simulink model "Q53"  (R2023a)
settings: Solver=VariableStepAuto  StartTime=0.0  StopTime=10.0  MaxStep=0.001  RelTol=1e-3
settings Model: Creator=Physics Library  LastModifiedBy=Physics Library

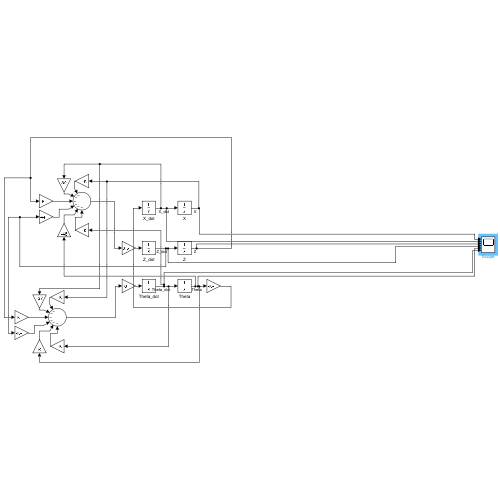
[thumbnail: Simulink's stored preview of the top-level diagram]
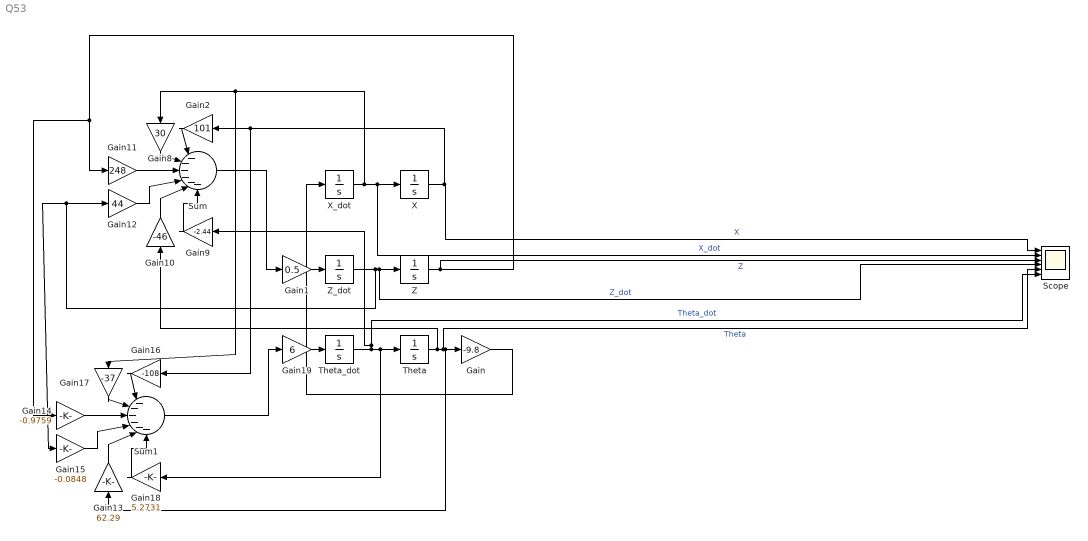
== system Q53 ==
  Gain : Gain  Gain=-9.8
  Gain1 : Gain  Gain=0.5
  Gain10 : Gain  Gain=-46
  Gain11 : Gain  Gain=248
  Gain12 : Gain  Gain=44
  Gain13 : Gain  Gain=62.29
  Gain14 : Gain  Gain=-0.9759
  Gain15 : Gain  Gain=-0.0848
  Gain16 : Gain  Gain=-108
  Gain17 : Gain  Gain=-37
  Gain18 : Gain  Gain=5.2731
  Gain19 : Gain  Gain=6
  Gain2 : Gain  Gain=101
  Gain8 : Gain  Gain=30
  Gain9 : Gain  Gain=-2.44
  Scope : Scope  NumInputPorts=6
  Sum : Sum  Inputs=|------
  Sum1 : Sum  Inputs=|------
  Theta : Integrator  InitialCondition=pi/6
  Theta_dot : Integrator
  X : Integrator
  X_dot : Integrator
  Z : Integrator  InitialCondition=1
  Z_dot : Integrator
  wires:
  Gain/1 -> X_dot/1
  X/1 -> Gain16/1, Gain2/1, Scope/1  "X"
  X_dot/1 -> Gain17/1, Gain8/1, X/1, Scope/2  "X_dot"
  Z/1 -> Scope/3, Gain14/1, Gain11/1  "Z"
  Z_dot/1 -> Gain12/1, Gain15/1, Scope/4, Z/1  "Z_dot"
  Theta/1 -> Gain10/1, Gain/1, Gain13/1, Scope/5  "Theta"
  Theta_dot/1 -> Gain18/1, Theta/1, Gain9/1, Scope/6  "Theta_dot"
  Gain2/1 -> Sum/1
  Gain8/1 -> Sum/2
  Gain9/1 -> Sum/6
  Gain10/1 -> Sum/5
  Gain11/1 -> Sum/3
  Gain12/1 -> Sum/4
  Gain1/1 -> Z_dot/1
  Sum/1 -> Gain1/1
  Gain15/1 -> Sum1/4
  Gain17/1 -> Sum1/2
  Gain18/1 -> Sum1/6
  Gain13/1 -> Sum1/5
  Sum1/1 -> Gain19/1
  Gain14/1 -> Sum1/3
  Gain16/1 -> Sum1/1
  Gain19/1 -> Theta_dot/1
